simulink model "ruidol"  (R2014b)
settings: Solver=ode45  StartTime=0.0  StopTime=100  RelTol=1e-3
libraries: simulink x1
settings Model: Creator=Permuta  LastModifiedBy=Permuta

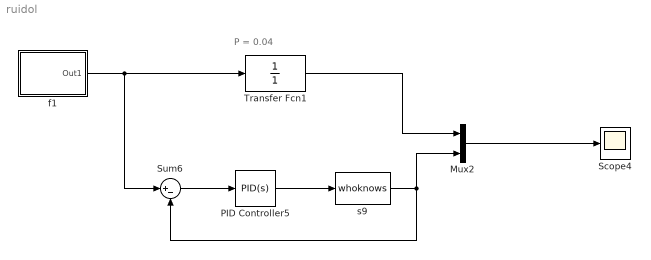
== system ruidol ==
  note: P = 0.04
  Mux2 : Mux  Inputs=2
  PID Controller5 : simulink/Continuous/PID Controller  Controller=PID  TimeDomain=Continuous-time  SampleTime=-1  IntegratorMethod=Forward Euler  FilterMethod=Forward Euler  Form=Parallel  P=0.048  I=0.0053333333  D=0.108  N=100  InitialConditionSource=internal  InitialConditionForIntegrator=0  InitialConditionForFilter=0  ExternalReset=none  LimitOutput=off  UpperSaturationLimit=inf  LowerSaturationLimit=-inf  LinearizeAsGain=on  AntiWindupMode=none  Kb=1  TrackingMode=off  Kt=1  PParamMin=[]  PParamMax=[]  IParamMin=[]  IParamMax=[]  DParamMin=[]  DParamMax=[]  NParamMin=[]  NParamMax=[]  KbParamMin=[]  KbParamMax=[]  KtParamMin=[]  KtParamMax=[]  POutMin=[]  POutMax=[]  IOutMin=[]  IOutMax=[]  DOutMin=[]  DOutMax=[]  NOutMin=[]  NOutMax=[]  KbOutMin=[]  KbOutMax=[]  KtOutMin=[]  KtOutMax=[]  IntegratorOutMin=[]  IntegratorOutMax=[]  FilterOutMin=[]  FilterOutMax=[]  SumOutMin=[]  SumOutMax=[]  SumI1OutMin=[]  SumI1OutMax=[]  SumI2OutMin=[]  SumI2OutMax=[]  SumI3OutMin=[]  SumI3OutMax=[]  SumDOutMin=[]  SumDOutMax=[]  SaturationOutMin=[]  SaturationOutMax=[]  IntegratorContinuousStateAttributes=''  IntegratorStateMustResolveToSignalObject=off  IntegratorRTWStateStorageClass=Auto  FilterContinuousStateAttributes=''  FilterStateMustResolveToSignalObject=off  FilterRTWStateStorageClass=Auto  DifferentiatorICPrevScaledInput=0  DifferentiatorOutMin=[]  DifferentiatorOutMax=[]  UseFilter=on
  Scope4 : Scope
      settings: TimeRange=10  YMin=-3  YMax=3  SaveName=Parte3
  Sum6 : Sum  Inputs=|+-
  Transfer Fcn1 : TransferFcn  Denominator=[0 1]
  f1 : Subsystem  mask{S=1, L=0, T=100}
      mask prompts: S "Limite Superior"; L "Limite Inferior"; T "Periodo de cambio"
      mask Display: disp('Ent. Variable')
  s9 : M-S-Function  FunctionName=whoknows  Parameters=L, P1, P2, T, R  mask{L=7, P1=0, P2=2, T=2, R=0.05}
      mask prompts: L "Laboratorio"; P1 "Primer digito del Puesto"; P2 "Segundo digito del Puesto"; T "Tipo de Planta"; R "Ruido"
      mask Display: disp('Sistema')
  wires:
  f1/1(Out1) -> Transfer Fcn1/1, Sum6/1
  s9/1 -> Sum6/2, Mux2/2
  PID Controller5/1 -> s9/1
  Sum6/1 -> PID Controller5/1
  Mux2/1 -> Scope4/1
  Transfer Fcn1/1 -> Mux2/1

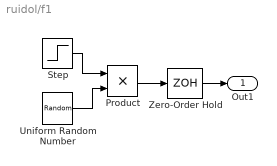
== system ruidol/f1 ==
  Product : Product  RndMeth=Zero
  Step : Step  Time=0  SampleTime=0
  Uniform Random Number : UniformRandomNumber  Minimum=L  Maximum=S  SampleTime=0
  Zero-Order Hold : ZeroOrderHold  SampleTime=T
  Out1 : Outport
  wires:
  Step/1 -> Product/1
  Uniform Random Number/1 -> Product/2
  Product/1 -> Zero-Order Hold/1
  Zero-Order Hold/1 -> Out1/1
